simulink model "tyreModelSimu"  (R2020b)
settings: Solver=VariableStepAuto  StartTime=0.0  StopTime=10.0  RelTol=1e-3
values from neighbouring files (symbols this model uses):
  h = 0.3    [Copy_of_model1.m]    (also in model1.m; test.m; tyreModel.m)
  l = lf+lr    (= 2)    [Copy_of_model1.m]    (also in model1.m; test.m = 1.5; tyreModel.m = 1.5)
  lf = 1    [Copy_of_model1.m]    (also in model1.m; test.m; tyreModel.m)
  lr = 1    [Copy_of_model1.m]    (also in model1.m; test.m = 0.5; tyreModel.m = 0.5)
  m = 200    [Copy_of_model1.m]    (also in model1.m; test.m; tyreModel.m)
  rsd = 0.25    [Copy_of_model1.m]    (also in model1.m; test.m; tyreModel.m)
  s1 = 0.5    [Copy_of_model1.m]    (also in model1.m; test.m; tyreModel.m = 1)
  s2 = 0    [Copy_of_model1.m]    (also in model1.m; test.m; tyreModel.m)
undefined symbols (not defined in the file or in its folder): p
libraries: vrlib x3
settings Model: Creator=picku  LastModifiedBy=picku

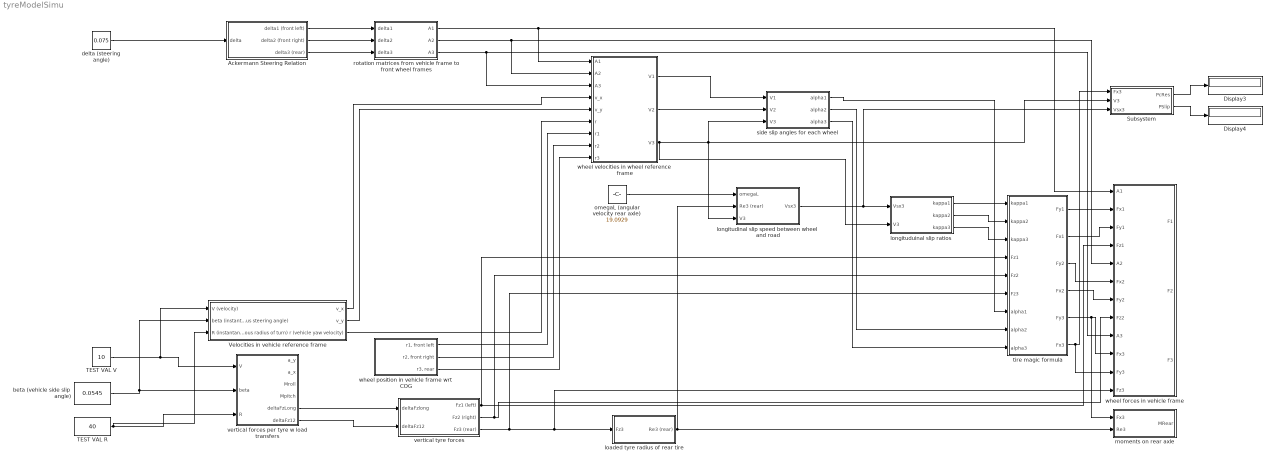
== system tyreModelSimu ==
  Ackermann Steering Relation : Subsystem
  Display3 : Display
  Display4 : Display
  Subsystem : Subsystem
  TEST VAL R : Constant  Value=40
  TEST VAL V : Constant  Value=10
  Velocities in vehicle reference frame : Subsystem
  beta (vehicle side slip angle) : Constant  Value=0.0545
  delta (steering angle) : Constant  Value=0.075
  loaded tyre radius of rear tire : Subsystem
  longitudinal slip speed between wheel and road : Subsystem
  longituduinal slip ratios : Subsystem
  moments on rear axle : Subsystem
  omegaL (angular velocity rear axle) : Constant  Value=19.0929
  rotation matrices from vehicle frame to front wheel frames : Subsystem
  side slip angles for each wheel : Subsystem
  tire magic formula : Subsystem
  vertical forces per tyre w load transfers : Subsystem
  vertical tyre forces : Subsystem
  wheel forces in vehicle frame : Subsystem
  wheel position in vehicle frame wrt COG : Subsystem
  wheel velocities in wheel reference frame : Subsystem
  wires:
  tire magic formula/6("Fx3 ") -> Subsystem/1(Fx3), wheel forces in vehicle frame/11(Fy3)
  longituduinal slip ratios/3(kappa3) -> tire magic formula/3(kappa3)
  tire magic formula/5(Fy3) -> wheel forces in vehicle frame/10(Fx3), moments on rear axle/1(Fx3)
  side slip angles for each wheel/3(alpha3) -> tire magic formula/9(alpha3)
  side slip angles for each wheel/1(alpha1) -> tire magic formula/7(alpha1)
  side slip angles for each wheel/2(alpha2) -> tire magic formula/8(alpha2)
  vertical tyre forces/1(Fz1 (left)) -> tire magic formula/4(Fz1), wheel forces in vehicle frame/4(Fz1)
  tire magic formula/1(Fy1) -> wheel forces in vehicle frame/2(Fx1)
  tire magic formula/2(Fx1) -> wheel forces in vehicle frame/3(Fy1)
  vertical tyre forces/2(Fz2 (right)) -> tire magic formula/5(Fz2), wheel forces in vehicle frame/8(Fz2)
  longituduinal slip ratios/1(kappa1) -> tire magic formula/1(kappa1)
  tire magic formula/4(Fx2) -> wheel forces in vehicle frame/7(Fy2)
  longituduinal slip ratios/2(kappa2) -> tire magic formula/2(kappa2)
  tire magic formula/3(Fy2) -> wheel forces in vehicle frame/6(Fx2)
  vertical tyre forces/3(Fz3 (rear)) -> loaded tyre radius of rear tire/1(Fz3), wheel forces in vehicle frame/12(Fz3), tire magic formula/6(Fz3)
  loaded tyre radius of rear tire/1(Re3 (rear)) -> moments on rear axle/2(Re3), longitudinal slip speed between wheel and road/2(Re3 (rear))
  wheel velocities in wheel reference frame/2(V2) -> side slip angles for each wheel/2(V2)
  longitudinal slip speed between wheel and road/1(Vsx3) -> Subsystem/3(Vsx3), longituduinal slip ratios/1(Vsx3)
  rotation matrices from vehicle frame to front wheel frames/3(A3) -> wheel velocities in wheel reference frame/3(A3), wheel forces in vehicle frame/9(A3)
  wheel position in vehicle frame wrt COG/2("r2, front right") -> wheel velocities in wheel reference frame/8(r2)
  vertical forces per tyre w load transfers/5(deltaFzLong) -> vertical tyre forces/1(deltaFzlong)
  omegaL (angular velocity rear axle)/1 -> longitudinal slip speed between wheel and road/1(omegaL)
  wheel position in vehicle frame wrt COG/3("r3, rear") -> wheel velocities in wheel reference frame/9(r3)
  wheel velocities in wheel reference frame/1(V1) -> side slip angles for each wheel/1(V1)
  vertical forces per tyre w load transfers/6(deltaFz12) -> vertical tyre forces/2(deltaFz12)
  Ackermann Steering Relation/1(delta1 (front left)) -> rotation matrices from vehicle frame to front wheel frames/1(delta1)
  wheel position in vehicle frame wrt COG/1("r1, front left") -> wheel velocities in wheel reference frame/7(r1)
  TEST VAL V/1 -> Velocities in vehicle reference frame/1(V (velocity)), vertical forces per tyre w load transfers/1(V)
  Velocities in vehicle reference frame/3(r (vehicle yaw velocity)) -> wheel velocities in wheel reference frame/6(r)
  rotation matrices from vehicle frame to front wheel frames/2(A2) -> wheel velocities in wheel reference frame/2(A2), wheel forces in vehicle frame/5(A2)
  wheel velocities in wheel reference frame/3(V3) -> side slip angles for each wheel/3(V3), Subsystem/2(V3), longitudinal slip speed between wheel and road/3(V3), longituduinal slip ratios/2(V3)
  Velocities in vehicle reference frame/1(v_x) -> wheel velocities in wheel reference frame/4(v_x)
  Velocities in vehicle reference frame/2(v_y) -> wheel velocities in wheel reference frame/5(v_y)
  rotation matrices from vehicle frame to front wheel frames/1(A1) -> wheel velocities in wheel reference frame/1(A1), wheel forces in vehicle frame/1(A1)
  Ackermann Steering Relation/3(delta3 (rear)) -> rotation matrices from vehicle frame to front wheel frames/3(delta3)
  Ackermann Steering Relation/2(delta2 (front right)) -> rotation matrices from vehicle frame to front wheel frames/2(delta2)
  delta (steering angle)/1 -> Ackermann Steering Relation/1(delta)
  TEST VAL R/1 -> Velocities in vehicle reference frame/3(R (instantaneous radius of turn)), vertical forces per tyre w load transfers/3(R)
  beta (vehicle side slip angle)/1 -> Velocities in vehicle reference frame/2(beta (instantaneous steering angle)), vertical forces per tyre w load transfers/2(beta)
  Subsystem/1(PcRes) -> Display3/1
  Subsystem/2(PSlip) -> Display4/1

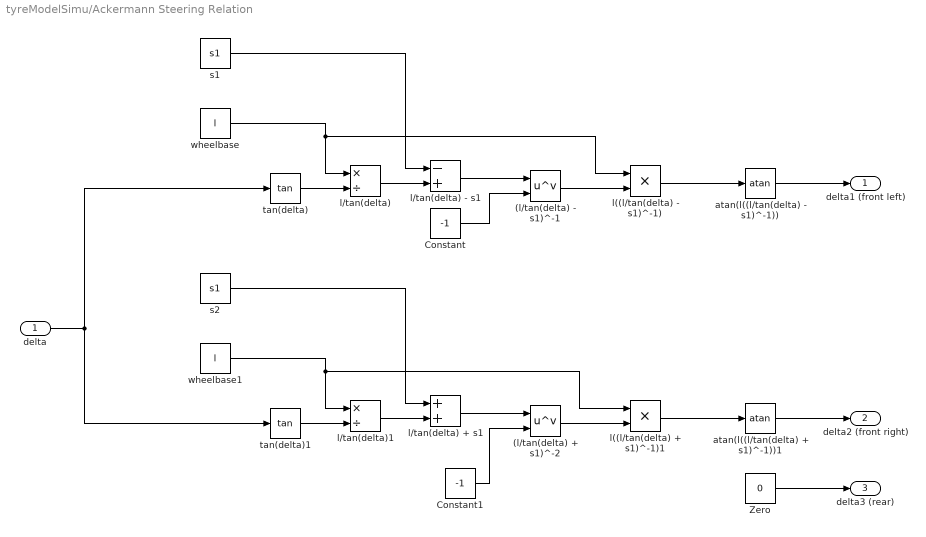
== system tyreModelSimu/Ackermann Steering Relation ==
  delta : Inport
  (l/tan(delta) + s1)^-2 : Math  Operator=pow  SaturateOnIntegerOverflow=on
  (l/tan(delta) - s1)^-1 : Math  Operator=pow  SaturateOnIntegerOverflow=on
  Constant : Constant  Value=-1
  Constant1 : Constant  Value=-1
  Zero : Constant  Value=0  OutDataTypeStr=Inherit: Inherit via back propagation
  atan(l((l/tan(delta) + s1)^-1))1 : Trigonometry  Operator=atan
  atan(l((l/tan(delta) - s1)^-1)) : Trigonometry  Operator=atan
  l((l/tan(delta) + s1)^-1)1 : Product
  l((l/tan(delta) - s1)^-1) : Product
  l/tan(delta) : Product  Inputs=*/
  l/tan(delta) + s1 : Sum
  l/tan(delta) - s1 : Sum  Inputs=-+
  l/tan(delta)1 : Product  Inputs=*/
  s1 : Constant  Value=s1
  s2 : Constant  Value=s1
  tan(delta) : Trigonometry  Operator=tan
  tan(delta)1 : Trigonometry  Operator=tan
  wheelbase : Constant  Value=l
  wheelbase1 : Constant  Value=l
  delta1 (front left) : Outport
  delta2 (front right) : Outport  Port=2
  delta3 (rear) : Outport  Port=3
  wires:
  tan(delta)/1 -> l/tan(delta)/2
  wheelbase/1 -> l((l/tan(delta) - s1)^-1)/1, l/tan(delta)/1
  l/tan(delta)/1 -> l/tan(delta) - s1/2
  s1/1 -> l/tan(delta) - s1/1
  l/tan(delta) - s1/1 -> (l/tan(delta) - s1)^-1/1
  Constant/1 -> (l/tan(delta) - s1)^-1/2
  (l/tan(delta) - s1)^-1/1 -> l((l/tan(delta) - s1)^-1)/2
  l((l/tan(delta) - s1)^-1)/1 -> atan(l((l/tan(delta) - s1)^-1))/1
  atan(l((l/tan(delta) - s1)^-1))/1 -> delta1 (front left)/1
  Constant1/1 -> (l/tan(delta) + s1)^-2/2
  wheelbase1/1 -> l((l/tan(delta) + s1)^-1)1/1, l/tan(delta)1/1
  tan(delta)1/1 -> l/tan(delta)1/2
  (l/tan(delta) + s1)^-2/1 -> l((l/tan(delta) + s1)^-1)1/2
  delta/1 -> tan(delta)1/1, tan(delta)/1
  l/tan(delta) + s1/1 -> (l/tan(delta) + s1)^-2/1
  l/tan(delta)1/1 -> l/tan(delta) + s1/2
  atan(l((l/tan(delta) + s1)^-1))1/1 -> delta2 (front right)/1
  l((l/tan(delta) + s1)^-1)1/1 -> atan(l((l/tan(delta) + s1)^-1))1/1
  s2/1 -> l/tan(delta) + s1/1
  Zero/1 -> delta3 (rear)/1

== system tyreModelSimu/Subsystem ==
  Fx3 : Inport
  V3 : Inport  Port=2
  Vsx3 : Inport  Port=3
  Demux : Demux  Outputs=3
  Product : Product
  Product1 : Product
  PcRes : Outport
  PSlip : Outport  Port=2
  wires:
  V3/1 -> Demux/1
  Demux/1 -> Product/2
  Fx3/1 -> Product1/2, Product/1
  Product/1 -> PcRes/1
  Vsx3/1 -> Product1/1
  Product1/1 -> PSlip/1

== system tyreModelSimu/Velocities in vehicle reference frame ==
  V (velocity) : Inport
  beta (instantaneous steering angle) : Inport  Port=2
  R (instantaneous radius of turn) : Inport  Port=3
  -V*sin(beta) : Product
  -sin(beta) : UnaryMinus
  Divide : Product  Inputs=*/
  V*cos(beta) : Product
  cos(beta) : Trigonometry  Operator=cos
  sin(beta) : Trigonometry
  v_x : Outport
  v_y : Outport  Port=2
  r (vehicle yaw velocity) : Outport  Port=3
  wires:
  beta (instantaneous steering angle)/1 -> sin(beta)/1, cos(beta)/1
  sin(beta)/1 -> -sin(beta)/1
  -sin(beta)/1 -> -V*sin(beta)/2
  V (velocity)/1 -> Divide/1, V*cos(beta)/1, -V*sin(beta)/1
  cos(beta)/1 -> V*cos(beta)/2
  -V*sin(beta)/1 -> v_y/1
  V*cos(beta)/1 -> v_x/1
  R (instantaneous radius of turn)/1 -> Divide/2
  Divide/1 -> r (vehicle yaw velocity)/1

== system tyreModelSimu/loaded tyre radius of rear tire ==
  Fz3 : Inport
  Display : Display
  Divide : Product  Inputs=*/
  Subtract : Sum  Inputs=-+
  free tyre radius : Constant  Value=p.tyre1.R0
  tyre vertical stiffness : Constant  Value=p.tyre1.kz
  Re3 (rear) : Outport
  wires:
  tyre vertical stiffness/1 -> Divide/2
  Fz3/1 -> Display/1, Divide/1
  Divide/1 -> Subtract/1
  free tyre radius/1 -> Subtract/2
  Subtract/1 -> Re3 (rear)/1

== system tyreModelSimu/longitudinal slip speed between wheel and road ==
  omegaL : Inport
  Re3 (rear) : Inport  Port=2
  V3 : Inport  Port=3
  Demux : Demux  Outputs=3
  Display{,1..3} (4 alike) : Display
  Product : Product
  Subtract : Sum  Inputs=-+
  Unary Minus : UnaryMinus
  Vsx3 : Outport
  wires:
  V3/1 -> Display2/1, Demux/1
  omegaL/1 -> Display/1, Product/1
  Re3 (rear)/1 -> Display1/1, Product/2
  Product/1 -> Subtract/1
  Demux/1 -> Subtract/2
  Subtract/1 -> Unary Minus/1
  Unary Minus/1 -> Display3/1, Vsx3/1

== system tyreModelSimu/longituduinal slip ratios ==
  Vsx3 : Inport
  V3 : Inport  Port=2
  Abs : Abs
  Demux : Demux  Outputs=3
  Divide : Product  Inputs=*/
  Zero : Constant  Value=0  OutDataTypeStr=Inherit: Inherit via back propagation
  kappa1 : Outport
  kappa2 : Outport  Port=2
  kappa3 : Outport  Port=3
  wires:
  Zero/1 -> kappa2/1, kappa1/1
  V3/1 -> Demux/1
  Demux/1 -> Abs/1
  Abs/1 -> Divide/2
  Vsx3/1 -> Divide/1
  Divide/1 -> kappa3/1

== system tyreModelSimu/moments on rear axle ==
  Fx3 : Inport
  Re3 : Inport  Port=2
  Product : Product
  MRear : Outport
  wires:
  Re3/1 -> Product/2
  Fx3/1 -> Product/1
  Product/1 -> MRear/1

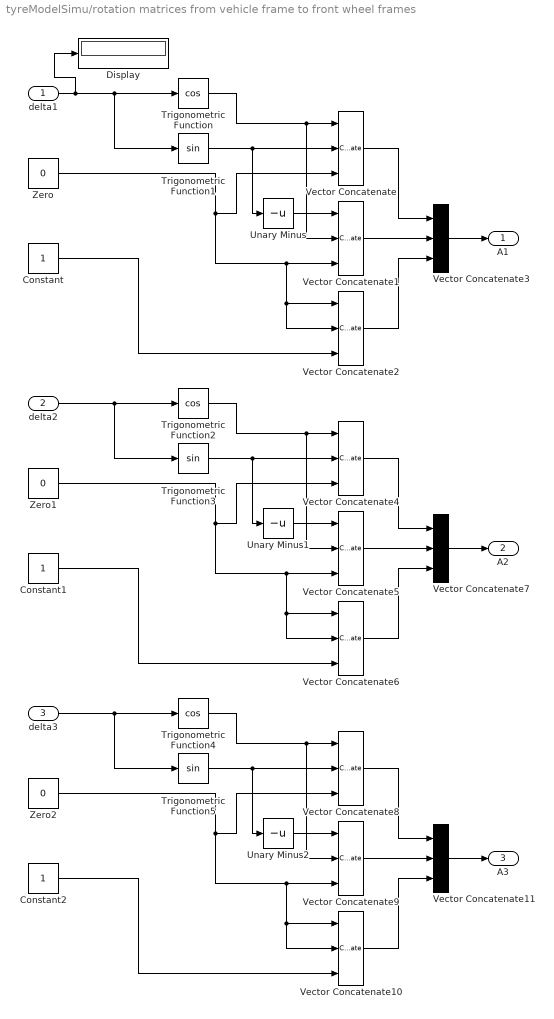
== system tyreModelSimu/rotation matrices from vehicle frame to front wheel frames ==
  delta1 : Inport
  delta2 : Inport  Port=2
  delta3 : Inport  Port=3
  Constant : Constant
  Constant1 : Constant
  Constant2 : Constant
  Display : Display
  Trigonometric Function : Trigonometry  Operator=cos
  Trigonometric Function1 : Trigonometry
  Trigonometric Function2 : Trigonometry  Operator=cos
  Trigonometric Function3 : Trigonometry
  Trigonometric Function4 : Trigonometry  Operator=cos
  Trigonometric Function5 : Trigonometry
  Unary Minus : UnaryMinus
  Unary Minus1 : UnaryMinus
  Unary Minus2 : UnaryMinus
  Vector Concatenate{,1..2,4..6,8..10} (9 alike) : Concatenate  NumInputs=3  Mode=Multidimensional array  ConcatenateDimension=2
  Vector Concatenate11 : Concatenate  NumInputs=3  Mode=Multidimensional array
  Vector Concatenate3 : Concatenate  NumInputs=3  Mode=Multidimensional array
  Vector Concatenate7 : Concatenate  NumInputs=3  Mode=Multidimensional array
  Zero : Constant  Value=0  OutDataTypeStr=Inherit: Inherit via back propagation
  Zero1 : Constant  Value=0  OutDataTypeStr=Inherit: Inherit via back propagation
  Zero2 : Constant  Value=0  OutDataTypeStr=Inherit: Inherit via back propagation
  A1 : Outport
  A2 : Outport  Port=2
  A3 : Outport  Port=3
  wires:
  delta1/1 -> Display/1, Trigonometric Function1/1, Trigonometric Function/1
  Trigonometric Function/1 -> Vector Concatenate1/2, Vector Concatenate/1
  Trigonometric Function1/1 -> Unary Minus/1, Vector Concatenate/2
  Zero/1 -> Vector Concatenate2/2, Vector Concatenate2/1, Vector Concatenate1/3, Vector Concatenate/3
  Unary Minus/1 -> Vector Concatenate1/1
  Constant/1 -> Vector Concatenate2/3
  Vector Concatenate/1 -> Vector Concatenate3/1
  Vector Concatenate1/1 -> Vector Concatenate3/2
  Vector Concatenate2/1 -> Vector Concatenate3/3
  Vector Concatenate3/1 -> A1/1
  Vector Concatenate7/1 -> A2/1
  Constant1/1 -> Vector Concatenate6/3
  Zero1/1 -> Vector Concatenate6/2, Vector Concatenate6/1, Vector Concatenate5/3, Vector Concatenate4/3
  Vector Concatenate5/1 -> Vector Concatenate7/2
  Vector Concatenate4/1 -> Vector Concatenate7/1
  Trigonometric Function2/1 -> Vector Concatenate5/2, Vector Concatenate4/1
  Trigonometric Function3/1 -> Unary Minus1/1, Vector Concatenate4/2
  delta2/1 -> Trigonometric Function3/1, Trigonometric Function2/1
  Vector Concatenate6/1 -> Vector Concatenate7/3
  Unary Minus1/1 -> Vector Concatenate5/1
  Vector Concatenate11/1 -> A3/1
  Constant2/1 -> Vector Concatenate10/3
  Zero2/1 -> Vector Concatenate10/2, Vector Concatenate10/1, Vector Concatenate9/3, Vector Concatenate8/3
  Vector Concatenate9/1 -> Vector Concatenate11/2
  Vector Concatenate8/1 -> Vector Concatenate11/1
  Trigonometric Function4/1 -> Vector Concatenate9/2, Vector Concatenate8/1
  Trigonometric Function5/1 -> Unary Minus2/1, Vector Concatenate8/2
  delta3/1 -> Trigonometric Function5/1, Trigonometric Function4/1
  Vector Concatenate10/1 -> Vector Concatenate11/3
  Unary Minus2/1 -> Vector Concatenate9/1

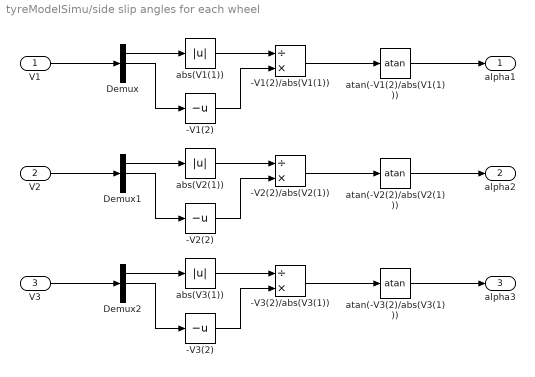
== system tyreModelSimu/side slip angles for each wheel ==
  V1 : Inport
  V2 : Inport  Port=2
  V3 : Inport  Port=3
  -V1(2) : UnaryMinus
  -V1(2)/abs(V1(1)) : Product  Inputs=/*
  -V2(2) : UnaryMinus
  -V2(2)/abs(V2(1)) : Product  Inputs=/*
  -V3(2) : UnaryMinus
  -V3(2)/abs(V3(1)) : Product  Inputs=/*
  Demux : Demux  Outputs=3
  Demux1 : Demux  Outputs=3
  Demux2 : Demux  Outputs=3
  abs(V1(1)) : Abs
  abs(V2(1)) : Abs
  abs(V3(1)) : Abs
  atan(-V1(2)/abs(V1(1))) : Trigonometry  Operator=atan
  atan(-V2(2)/abs(V2(1))) : Trigonometry  Operator=atan
  atan(-V3(2)/abs(V3(1))) : Trigonometry  Operator=atan
  alpha1 : Outport
  alpha2 : Outport  Port=2
  alpha3 : Outport  Port=3
  wires:
  V1/1 -> Demux/1
  Demux/1 -> abs(V1(1))/1
  Demux/2 -> -V1(2)/1
  abs(V1(1))/1 -> -V1(2)/abs(V1(1))/1
  -V1(2)/1 -> -V1(2)/abs(V1(1))/2
  -V1(2)/abs(V1(1))/1 -> atan(-V1(2)/abs(V1(1)))/1
  atan(-V1(2)/abs(V1(1)))/1 -> alpha1/1
  abs(V2(1))/1 -> -V2(2)/abs(V2(1))/1
  -V2(2)/1 -> -V2(2)/abs(V2(1))/2
  Demux1/2 -> -V2(2)/1
  -V2(2)/abs(V2(1))/1 -> atan(-V2(2)/abs(V2(1)))/1
  V2/1 -> Demux1/1
  Demux1/1 -> abs(V2(1))/1
  atan(-V2(2)/abs(V2(1)))/1 -> alpha2/1
  abs(V3(1))/1 -> -V3(2)/abs(V3(1))/1
  -V3(2)/1 -> -V3(2)/abs(V3(1))/2
  Demux2/2 -> -V3(2)/1
  -V3(2)/abs(V3(1))/1 -> atan(-V3(2)/abs(V3(1)))/1
  V3/1 -> Demux2/1
  Demux2/1 -> abs(V3(1))/1
  atan(-V3(2)/abs(V3(1)))/1 -> alpha3/1

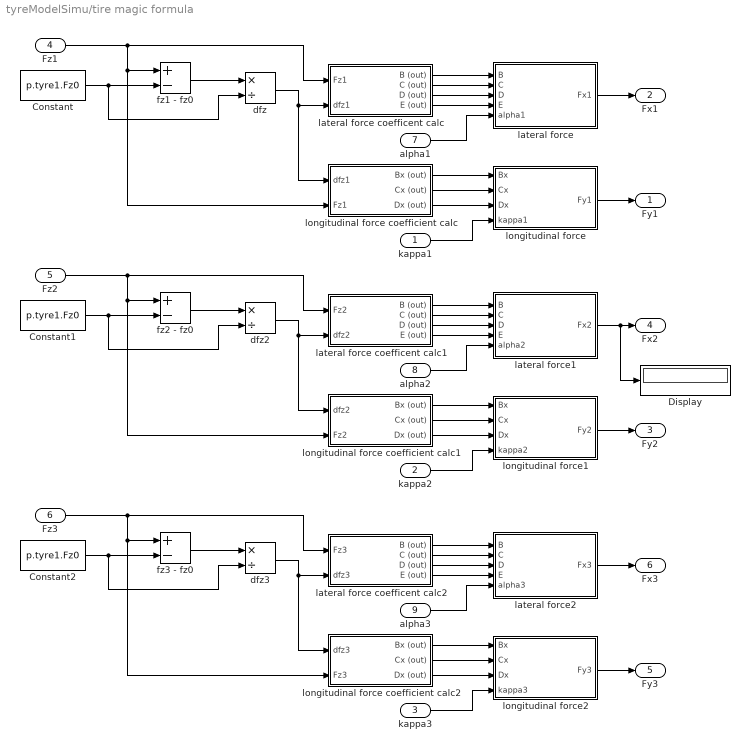
== system tyreModelSimu/tire magic formula ==
  kappa1 : Inport
  kappa2 : Inport  Port=2
  kappa3 : Inport  Port=3
  Fz1 : Inport  Port=4
  Fz2 : Inport  Port=5
  Fz3 : Inport  Port=6
  alpha1 : Inport  Port=7
  alpha2 : Inport  Port=8
  alpha3 : Inport  Port=9
  Constant : Constant  Value=p.tyre1.Fz0
  Constant1 : Constant  Value=p.tyre1.Fz0
  Constant2 : Constant  Value=p.tyre1.Fz0
  Display : Display
  dfz : Product  Inputs=*/
  dfz2 : Product  Inputs=*/
  dfz3 : Product  Inputs=*/
  fz1 - fz0 : Sum  Inputs=+-
  fz2 - fz0 : Sum  Inputs=+-
  fz3 - fz0 : Sum  Inputs=+-
  lateral force : Subsystem
  lateral force coefficent calc : Subsystem
  lateral force coefficent calc1 : Subsystem
  lateral force coefficent calc2 : Subsystem
  lateral force1 : Subsystem
  lateral force2 : Subsystem
  longitudinal force : Subsystem
  longitudinal force coefficient calc : Subsystem
  longitudinal force coefficient calc1 : Subsystem
  longitudinal force coefficient calc2 : Subsystem
  longitudinal force1 : Subsystem
  longitudinal force2 : Subsystem
  Fy1 : Outport
  Fx1 : Outport  Port=2
  Fy2 : Outport  Port=3
  Fx2 : Outport  Port=4
  Fy3 : Outport  Port=5
  "Fx3 " : Outport  Port=6
  wires:
  Fz1/1 -> lateral force coefficent calc/1(Fz1), longitudinal force coefficient calc/2(Fz1), fz1 - fz0/1
  Constant/1 -> fz1 - fz0/2, dfz/2
  fz1 - fz0/1 -> dfz/1
  dfz/1 -> longitudinal force coefficient calc/1(dfz1), lateral force coefficent calc/2(dfz1)
  lateral force coefficent calc/1(B (out)) -> lateral force/1(B)
  lateral force coefficent calc/2(C (out)) -> lateral force/2(C)
  lateral force coefficent calc/3(D (out)) -> lateral force/3(D)
  lateral force coefficent calc/4(E (out)) -> lateral force/4(E)
  alpha1/1 -> lateral force/5(alpha1)
  kappa1/1 -> longitudinal force/4(kappa1)
  longitudinal force coefficient calc/1(Bx (out)) -> longitudinal force/1(Bx)
  longitudinal force coefficient calc/2(Cx (out)) -> longitudinal force/2(Cx)
  longitudinal force coefficient calc/3(Dx (out)) -> longitudinal force/3(Dx)
  lateral force coefficent calc1/3(D (out)) -> lateral force1/3(D)
  lateral force coefficent calc1/4(E (out)) -> lateral force1/4(E)
  lateral force coefficent calc1/2(C (out)) -> lateral force1/2(C)
  longitudinal force coefficient calc1/2(Cx (out)) -> longitudinal force1/2(Cx)
  alpha2/1 -> lateral force1/5(alpha2)
  longitudinal force coefficient calc1/3(Dx (out)) -> longitudinal force1/3(Dx)
  longitudinal force coefficient calc1/1(Bx (out)) -> longitudinal force1/1(Bx)
  Fz2/1 -> lateral force coefficent calc1/1(Fz2), longitudinal force coefficient calc1/2(Fz2), fz2 - fz0/1
  fz2 - fz0/1 -> dfz2/1
  Constant1/1 -> fz2 - fz0/2, dfz2/2
  dfz2/1 -> longitudinal force coefficient calc1/1(dfz2), lateral force coefficent calc1/2(dfz2)
  kappa2/1 -> longitudinal force1/4(kappa2)
  lateral force coefficent calc1/1(B (out)) -> lateral force1/1(B)
  lateral force coefficent calc2/3(D (out)) -> lateral force2/3(D)
  lateral force coefficent calc2/4(E (out)) -> lateral force2/4(E)
  lateral force coefficent calc2/2(C (out)) -> lateral force2/2(C)
  longitudinal force coefficient calc2/2(Cx (out)) -> longitudinal force2/2(Cx)
  alpha3/1 -> lateral force2/5(alpha3)
  longitudinal force coefficient calc2/3(Dx (out)) -> longitudinal force2/3(Dx)
  longitudinal force coefficient calc2/1(Bx (out)) -> longitudinal force2/1(Bx)
  Fz3/1 -> lateral force coefficent calc2/1(Fz3), longitudinal force coefficient calc2/2(Fz3), fz3 - fz0/1
  fz3 - fz0/1 -> dfz3/1
  Constant2/1 -> fz3 - fz0/2, dfz3/2
  dfz3/1 -> longitudinal force coefficient calc2/1(dfz3), lateral force coefficent calc2/2(dfz3)
  kappa3/1 -> longitudinal force2/4(kappa3)
  lateral force coefficent calc2/1(B (out)) -> lateral force2/1(B)
  longitudinal force/1(Fy1) -> Fy1/1
  lateral force/1(Fx1) -> Fx1/1
  longitudinal force1/1(Fy2) -> Fy2/1
  lateral force1/1(Fx2) -> Display/1, Fx2/1
  longitudinal force2/1(Fy3) -> Fy3/1
  lateral force2/1(Fx3) -> "Fx3 "/1

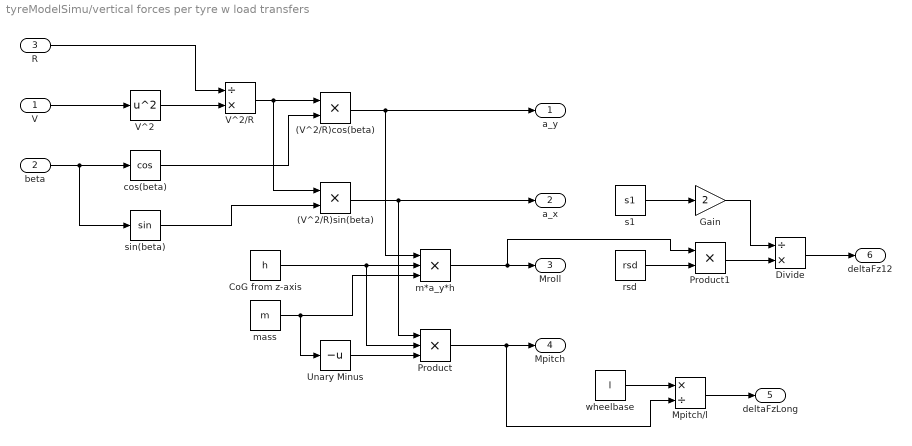
== system tyreModelSimu/vertical forces per tyre w load transfers ==
  V : Inport
  beta : Inport  Port=2
  R : Inport  Port=3
  (V^2/R)cos(beta) : Product
  (V^2/R)sin(beta) : Product
  CoG from z-axis : Constant  Value=h
  Divide : Product  Inputs=/*
  Gain : Gain  Gain=2
  Mpitch/l : Product  Inputs=*/
  Product : Product  Inputs=3
  Product1 : Product
  Unary Minus : UnaryMinus
  V^2 : Math  Operator=square  SaturateOnIntegerOverflow=on
  V^2/R : Product  Inputs=/*
  cos(beta) : Trigonometry  Operator=cos
  m*a_y*h : Product  Inputs=3
  mass : Constant  Value=m
  rsd : Constant  Value=rsd
  s1 : Constant  Value=s1
  sin(beta) : Trigonometry
  wheelbase : Constant  Value=l
  a_y : Outport
  a_x : Outport  Port=2
  Mroll : Outport  Port=3
  Mpitch : Outport  Port=4
  deltaFzLong : Outport  Port=5
  deltaFz12 : Outport  Port=6
  wires:
  V/1 -> V^2/1
  R/1 -> V^2/R/1
  V^2/1 -> V^2/R/2
  beta/1 -> sin(beta)/1, cos(beta)/1
  V^2/R/1 -> (V^2/R)sin(beta)/1, (V^2/R)cos(beta)/1
  cos(beta)/1 -> (V^2/R)cos(beta)/2
  (V^2/R)cos(beta)/1 -> m*a_y*h/1, a_y/1
  sin(beta)/1 -> (V^2/R)sin(beta)/2
  (V^2/R)sin(beta)/1 -> Product/1, a_x/1
  CoG from z-axis/1 -> Product/2, m*a_y*h/2
  mass/1 -> Unary Minus/1, m*a_y*h/3
  m*a_y*h/1 -> Product1/1, Mroll/1
  Product/1 -> Mpitch/l/2, Mpitch/1
  Unary Minus/1 -> Product/3
  wheelbase/1 -> Mpitch/l/1
  Mpitch/l/1 -> deltaFzLong/1
  rsd/1 -> Product1/2
  s1/1 -> Gain/1
  Product1/1 -> Divide/2
  Gain/1 -> Divide/1
  Divide/1 -> deltaFz12/1

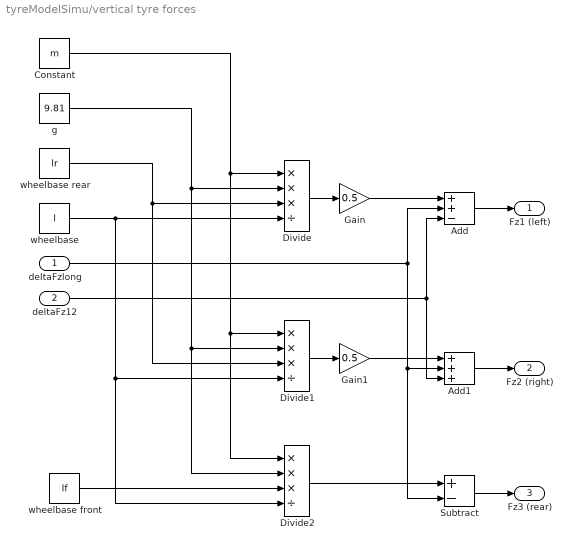
== system tyreModelSimu/vertical tyre forces ==
  deltaFzlong : Inport
  deltaFz12 : Inport  Port=2
  Add : Sum  Inputs=++-
  Add1 : Sum  Inputs=+++
  Constant : Constant  Value=m
  Divide : Product  Inputs=***/
  Divide1 : Product  Inputs=***/
  Divide2 : Product  Inputs=***/
  Gain : Gain  Gain=0.5
  Gain1 : Gain  Gain=0.5
  Subtract : Sum  Inputs=+-
  g : Constant  Value=9.81
  wheelbase : Constant  Value=l
  wheelbase front : Constant  Value=lf
  wheelbase rear : Constant  Value=lr
  Fz1 (left) : Outport
  Fz2 (right) : Outport  Port=2
  Fz3 (rear) : Outport  Port=3
  wires:
  Constant/1 -> Divide2/1, Divide1/1, Divide/1
  g/1 -> Divide2/2, Divide1/2, Divide/2
  wheelbase rear/1 -> Divide1/3, Divide/3
  wheelbase/1 -> Divide2/4, Divide1/4, Divide/4
  Divide/1 -> Gain/1
  Gain/1 -> Add/1
  deltaFzlong/1 -> Subtract/2, Add1/2, Add/2
  deltaFz12/1 -> Add1/3, Add/3
  Add/1 -> Fz1 (left)/1
  Gain1/1 -> Add1/1
  Add1/1 -> Fz2 (right)/1
  Divide1/1 -> Gain1/1
  wheelbase front/1 -> Divide2/3
  Divide2/1 -> Subtract/1
  Subtract/1 -> Fz3 (rear)/1

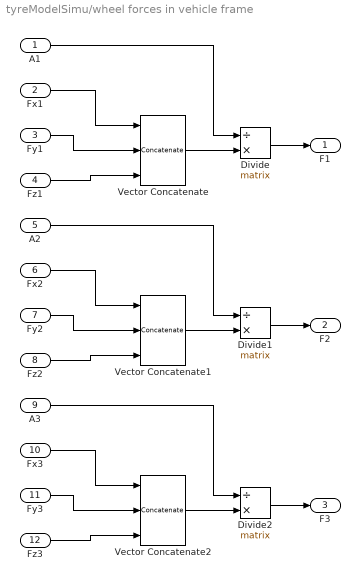
== system tyreModelSimu/wheel forces in vehicle frame ==
  A1 : Inport
  Fx1 : Inport  Port=2
  Fy1 : Inport  Port=3
  Fz1 : Inport  Port=4
  A2 : Inport  Port=5
  Fx2 : Inport  Port=6
  Fy2 : Inport  Port=7
  Fz2 : Inport  Port=8
  A3 : Inport  Port=9
  Fx3 : Inport  Port=10
  Fy3 : Inport  Port=11
  Fz3 : Inport  Port=12
  Divide : Product  Inputs=/*  Multiplication=Matrix(*)
  Divide1 : Product  Inputs=/*  Multiplication=Matrix(*)
  Divide2 : Product  Inputs=/*  Multiplication=Matrix(*)
  Vector Concatenate : Concatenate  NumInputs=3  Mode=Multidimensional array
  Vector Concatenate1 : Concatenate  NumInputs=3  Mode=Multidimensional array
  Vector Concatenate2 : Concatenate  NumInputs=3  Mode=Multidimensional array
  F1 : Outport
  F2 : Outport  Port=2
  F3 : Outport  Port=3
  wires:
  Fx1/1 -> Vector Concatenate/1
  Fy1/1 -> Vector Concatenate/2
  Fz1/1 -> Vector Concatenate/3
  Vector Concatenate/1 -> Divide/2
  A1/1 -> Divide/1
  Divide/1 -> F1/1
  Fz2/1 -> Vector Concatenate1/3
  Divide1/1 -> F2/1
  A2/1 -> Divide1/1
  Fy2/1 -> Vector Concatenate1/2
  Vector Concatenate1/1 -> Divide1/2
  Fx2/1 -> Vector Concatenate1/1
  Fz3/1 -> Vector Concatenate2/3
  Divide2/1 -> F3/1
  A3/1 -> Divide2/1
  Fy3/1 -> Vector Concatenate2/2
  Vector Concatenate2/1 -> Divide2/2
  Fx3/1 -> Vector Concatenate2/1

== system tyreModelSimu/wheel position in vehicle frame wrt COG ==
  Unary Minus : UnaryMinus
  Unary Minus1 : UnaryMinus
  Zero : Constant  Value=0  OutDataTypeStr=Inherit: Inherit via back propagation
  front lateral axle length / 2 : Constant  Value=s1
  r1 front left : Concatenate  NumInputs=3  Mode=Multidimensional array
  r2 front right : Concatenate  NumInputs=3  Mode=Multidimensional array
  r3 rear : Concatenate  NumInputs=3  Mode=Multidimensional array
  rear lateral axle length : Constant  Value=s2
  wheelbase front : Constant  Value=lf
  wheelbase rear : Constant  Value=lr
  "r1, front left" : Outport
  "r2, front right" : Outport  Port=2
  "r3, rear" : Outport  Port=3
  wires:
  wheelbase front/1 -> r2 front right/1, r1 front left/1
  r1 front left/1 -> "r1, front left"/1
  front lateral axle length / 2/1 -> r1 front left/2, Unary Minus/1
  Zero/1 -> r2 front right/3, r3 rear/3, r1 front left/3
  Unary Minus/1 -> r2 front right/2
  r2 front right/1 -> "r2, front right"/1
  Unary Minus1/1 -> r3 rear/1
  wheelbase rear/1 -> Unary Minus1/1
  rear lateral axle length/1 -> r3 rear/2
  r3 rear/1 -> "r3, rear"/1

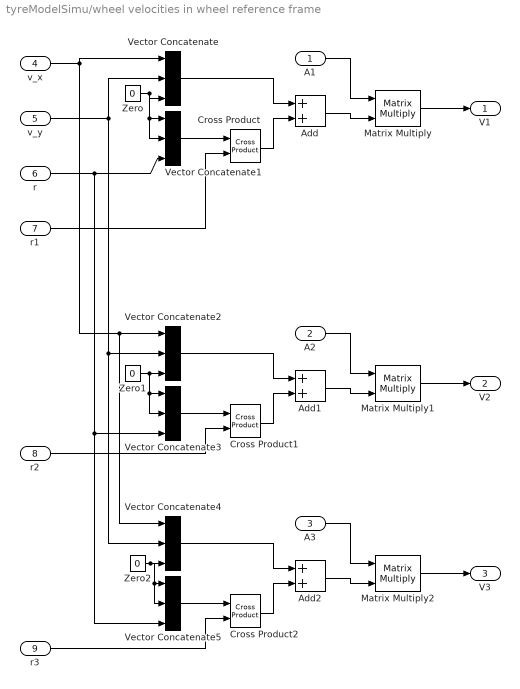
== system tyreModelSimu/wheel velocities in wheel reference frame ==
  A1 : Inport
  A2 : Inport  Port=2
  A3 : Inport  Port=3
  v_x : Inport  Port=4
  v_y : Inport  Port=5
  r : Inport  Port=6
  r1 : Inport  Port=7
  r2 : Inport  Port=8
  r3 : Inport  Port=9
  Add : Sum
  Add1 : Sum
  Add2 : Sum
  Cross Product : vrlib/Utilities/Cross Product
  Cross Product1 : vrlib/Utilities/Cross Product
  Cross Product2 : vrlib/Utilities/Cross Product
  Matrix Multiply : Product  Multiplication=Matrix(*)
  Matrix Multiply1 : Product  Multiplication=Matrix(*)
  Matrix Multiply2 : Product  Multiplication=Matrix(*)
  Vector Concatenate{,1..5} (6 alike) : Concatenate  NumInputs=3  Mode=Multidimensional array
  Zero : Constant  Value=0  OutDataTypeStr=Inherit: Inherit via back propagation
  Zero1 : Constant  Value=0  OutDataTypeStr=Inherit: Inherit via back propagation
  Zero2 : Constant  Value=0  OutDataTypeStr=Inherit: Inherit via back propagation
  V1 : Outport
  V2 : Outport  Port=2
  V3 : Outport  Port=3
  wires:
  Zero/1 -> Vector Concatenate1/2, Vector Concatenate1/1, Vector Concatenate/3
  Vector Concatenate1/1 -> Cross Product/1
  r1/1 -> Cross Product/2
  Cross Product/1 -> Add/2
  Vector Concatenate/1 -> Add/1
  Add/1 -> Matrix Multiply/2
  A1/1 -> Matrix Multiply/1
  Matrix Multiply/1 -> V1/1
  A2/1 -> Matrix Multiply1/1
  Matrix Multiply1/1 -> V2/1
  r2/1 -> Cross Product1/2
  Cross Product1/1 -> Add1/2
  r/1 -> Vector Concatenate1/3, Vector Concatenate5/3, Vector Concatenate3/3
  Vector Concatenate3/1 -> Cross Product1/1
  v_y/1 -> Vector Concatenate4/2, Vector Concatenate2/2, Vector Concatenate/2
  Zero1/1 -> Vector Concatenate2/3, Vector Concatenate3/2, Vector Concatenate3/1
  Add1/1 -> Matrix Multiply1/2
  Vector Concatenate2/1 -> Add1/1
  v_x/1 -> Vector Concatenate4/1, Vector Concatenate2/1, Vector Concatenate/1
  Vector Concatenate4/1 -> Add2/1
  Cross Product2/1 -> Add2/2
  Matrix Multiply2/1 -> V3/1
  Vector Concatenate5/1 -> Cross Product2/1
  Add2/1 -> Matrix Multiply2/2
  Zero2/1 -> Vector Concatenate5/1, Vector Concatenate5/2, Vector Concatenate4/3
  r3/1 -> Cross Product2/2
  A3/1 -> Matrix Multiply2/1

== system tyreModelSimu/tire magic formula/lateral force ==
  B : Inport
  C : Inport  Port=2
  D : Inport  Port=3
  E : Inport  Port=4
  alpha1 : Inport  Port=5
  " " : Product
  Add : Sum
  Constant : Constant
  Product : Product
  Product1 : Product
  Product2 : Product  Inputs=3
  Product3 : Product
  Subtract : Sum  Inputs=+-
  Trigonometric Function : Trigonometry  Operator=atan
  Trigonometric Function1 : Trigonometry  Operator=atan
  Trigonometric Function2 : Trigonometry
  Fx1 : Outport
  wires:
  alpha1/1 -> Subtract/2, Product2/2, Product/2
  B/1 -> Product/1, Product2/3
  Product/1 -> Trigonometric Function/1
  Trigonometric Function/1 -> Product1/2
  E/1 -> Product1/1
  Product1/1 -> Add/2
  Constant/1 -> Subtract/1
  Subtract/1 -> Product2/1
  Product2/1 -> Add/1
  Add/1 -> Trigonometric Function1/1
  Trigonometric Function1/1 -> Product3/2
  C/1 -> Product3/1
  Product3/1 -> Trigonometric Function2/1
  Trigonometric Function2/1 -> " "/2
  D/1 -> " "/1
  " "/1 -> Fx1/1

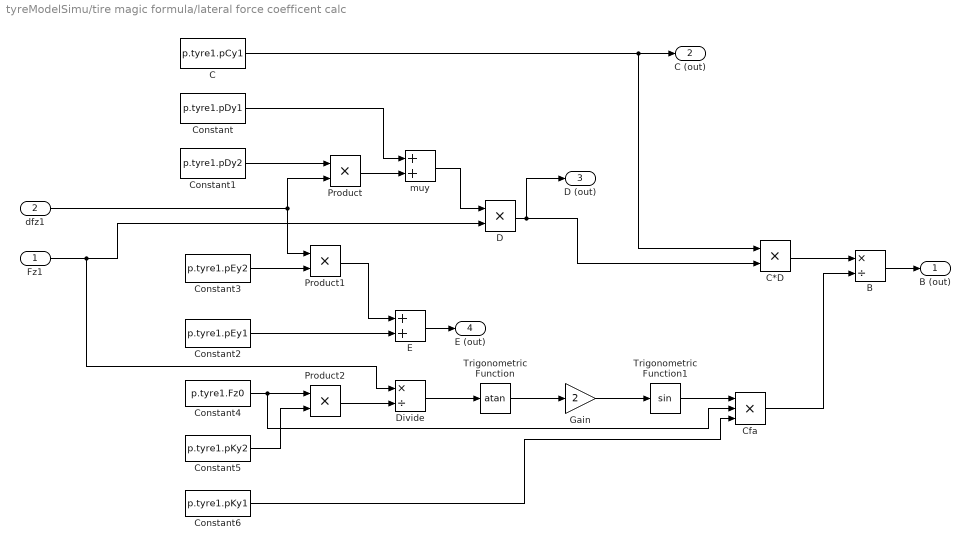
== system tyreModelSimu/tire magic formula/lateral force coefficent calc ==
  Fz1 : Inport
  dfz1 : Inport  Port=2
  B : Product  Inputs=*/
  C : Constant  Value=p.tyre1.pCy1
  C*D : Product
  Cfa : Product  Inputs=3
  Constant : Constant  Value=p.tyre1.pDy1
  Constant1 : Constant  Value=p.tyre1.pDy2
  Constant2 : Constant  Value=p.tyre1.pEy1
  Constant3 : Constant  Value=p.tyre1.pEy2
  Constant4 : Constant  Value=p.tyre1.Fz0
  Constant5 : Constant  Value=p.tyre1.pKy2
  Constant6 : Constant  Value=p.tyre1.pKy1
  D : Product
  Divide : Product  Inputs=*/
  E : Sum
  Gain : Gain  Gain=2
  Product : Product
  Product1 : Product
  Product2 : Product
  Trigonometric Function : Trigonometry  Operator=atan
  Trigonometric Function1 : Trigonometry
  muy : Sum
  B (out) : Outport
  C (out) : Outport  Port=2
  D (out) : Outport  Port=3
  E (out) : Outport  Port=4
  wires:
  dfz1/1 -> Product1/1, Product/2
  Constant1/1 -> Product/1
  Product/1 -> muy/2
  Constant/1 -> muy/1
  Fz1/1 -> Divide/1, D/2
  muy/1 -> D/1
  Constant3/1 -> Product1/2
  Product1/1 -> E/1
  Constant2/1 -> E/2
  Constant4/1 -> Product2/1, Cfa/2
  Constant5/1 -> Product2/2
  Product2/1 -> Divide/2
  Divide/1 -> Trigonometric Function/1
  Trigonometric Function/1 -> Gain/1
  Gain/1 -> Trigonometric Function1/1
  Trigonometric Function1/1 -> Cfa/1
  Constant6/1 -> Cfa/3
  C/1 -> C (out)/1, C*D/1
  D/1 -> D (out)/1, C*D/2
  C*D/1 -> B/1
  Cfa/1 -> B/2
  B/1 -> B (out)/1
  E/1 -> E (out)/1

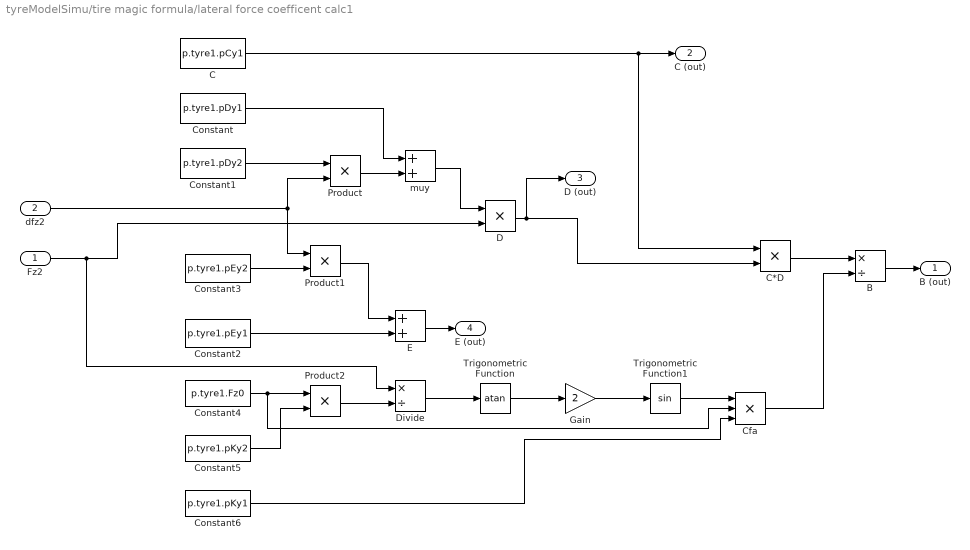
== system tyreModelSimu/tire magic formula/lateral force coefficent calc1 ==
  Fz2 : Inport
  dfz2 : Inport  Port=2
  B : Product  Inputs=*/
  C : Constant  Value=p.tyre1.pCy1
  C*D : Product
  Cfa : Product  Inputs=3
  Constant : Constant  Value=p.tyre1.pDy1
  Constant1 : Constant  Value=p.tyre1.pDy2
  Constant2 : Constant  Value=p.tyre1.pEy1
  Constant3 : Constant  Value=p.tyre1.pEy2
  Constant4 : Constant  Value=p.tyre1.Fz0
  Constant5 : Constant  Value=p.tyre1.pKy2
  Constant6 : Constant  Value=p.tyre1.pKy1
  D : Product
  Divide : Product  Inputs=*/
  E : Sum
  Gain : Gain  Gain=2
  Product : Product
  Product1 : Product
  Product2 : Product
  Trigonometric Function : Trigonometry  Operator=atan
  Trigonometric Function1 : Trigonometry
  muy : Sum
  B (out) : Outport
  C (out) : Outport  Port=2
  D (out) : Outport  Port=3
  E (out) : Outport  Port=4
  wires:
  dfz2/1 -> Product1/1, Product/2
  Constant1/1 -> Product/1
  Product/1 -> muy/2
  Constant/1 -> muy/1
  Fz2/1 -> Divide/1, D/2
  muy/1 -> D/1
  Constant3/1 -> Product1/2
  Product1/1 -> E/1
  Constant2/1 -> E/2
  Constant4/1 -> Product2/1, Cfa/2
  Constant5/1 -> Product2/2
  Product2/1 -> Divide/2
  Divide/1 -> Trigonometric Function/1
  Trigonometric Function/1 -> Gain/1
  Gain/1 -> Trigonometric Function1/1
  Trigonometric Function1/1 -> Cfa/1
  Constant6/1 -> Cfa/3
  C/1 -> C (out)/1, C*D/1
  D/1 -> D (out)/1, C*D/2
  C*D/1 -> B/1
  Cfa/1 -> B/2
  B/1 -> B (out)/1
  E/1 -> E (out)/1

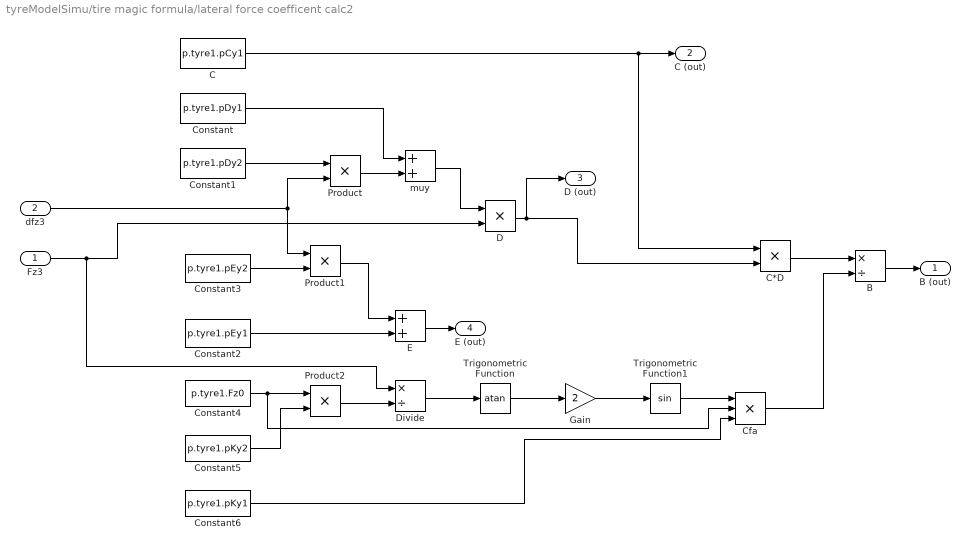
== system tyreModelSimu/tire magic formula/lateral force coefficent calc2 ==
  Fz3 : Inport
  dfz3 : Inport  Port=2
  B : Product  Inputs=*/
  C : Constant  Value=p.tyre1.pCy1
  C*D : Product
  Cfa : Product  Inputs=3
  Constant : Constant  Value=p.tyre1.pDy1
  Constant1 : Constant  Value=p.tyre1.pDy2
  Constant2 : Constant  Value=p.tyre1.pEy1
  Constant3 : Constant  Value=p.tyre1.pEy2
  Constant4 : Constant  Value=p.tyre1.Fz0
  Constant5 : Constant  Value=p.tyre1.pKy2
  Constant6 : Constant  Value=p.tyre1.pKy1
  D : Product
  Divide : Product  Inputs=*/
  E : Sum
  Gain : Gain  Gain=2
  Product : Product
  Product1 : Product
  Product2 : Product
  Trigonometric Function : Trigonometry  Operator=atan
  Trigonometric Function1 : Trigonometry
  muy : Sum
  B (out) : Outport
  C (out) : Outport  Port=2
  D (out) : Outport  Port=3
  E (out) : Outport  Port=4
  wires:
  dfz3/1 -> Product1/1, Product/2
  Constant1/1 -> Product/1
  Product/1 -> muy/2
  Constant/1 -> muy/1
  Fz3/1 -> Divide/1, D/2
  muy/1 -> D/1
  Constant3/1 -> Product1/2
  Product1/1 -> E/1
  Constant2/1 -> E/2
  Constant4/1 -> Product2/1, Cfa/2
  Constant5/1 -> Product2/2
  Product2/1 -> Divide/2
  Divide/1 -> Trigonometric Function/1
  Trigonometric Function/1 -> Gain/1
  Gain/1 -> Trigonometric Function1/1
  Trigonometric Function1/1 -> Cfa/1
  Constant6/1 -> Cfa/3
  C/1 -> C (out)/1, C*D/1
  D/1 -> D (out)/1, C*D/2
  C*D/1 -> B/1
  Cfa/1 -> B/2
  B/1 -> B (out)/1
  E/1 -> E (out)/1

== system tyreModelSimu/tire magic formula/lateral force1 ==
  B : Inport
  C : Inport  Port=2
  D : Inport  Port=3
  E : Inport  Port=4
  alpha2 : Inport  Port=5
  " " : Product
  Add : Sum
  Constant : Constant
  Product : Product
  Product1 : Product
  Product2 : Product  Inputs=3
  Product3 : Product
  Subtract : Sum  Inputs=+-
  Trigonometric Function : Trigonometry  Operator=atan
  Trigonometric Function1 : Trigonometry  Operator=atan
  Trigonometric Function2 : Trigonometry
  Fx2 : Outport
  wires:
  alpha2/1 -> Subtract/2, Product2/2, Product/2
  B/1 -> Product/1, Product2/3
  Product/1 -> Trigonometric Function/1
  Trigonometric Function/1 -> Product1/2
  E/1 -> Product1/1
  Product1/1 -> Add/2
  Constant/1 -> Subtract/1
  Subtract/1 -> Product2/1
  Product2/1 -> Add/1
  Add/1 -> Trigonometric Function1/1
  Trigonometric Function1/1 -> Product3/2
  C/1 -> Product3/1
  Product3/1 -> Trigonometric Function2/1
  Trigonometric Function2/1 -> " "/2
  D/1 -> " "/1
  " "/1 -> Fx2/1

== system tyreModelSimu/tire magic formula/lateral force2 ==
  B : Inport
  C : Inport  Port=2
  D : Inport  Port=3
  E : Inport  Port=4
  alpha3 : Inport  Port=5
  " " : Product
  Add : Sum
  Constant : Constant
  Product : Product
  Product1 : Product
  Product2 : Product  Inputs=3
  Product3 : Product
  Subtract : Sum  Inputs=+-
  Trigonometric Function : Trigonometry  Operator=atan
  Trigonometric Function1 : Trigonometry  Operator=atan
  Trigonometric Function2 : Trigonometry
  Fx3 : Outport
  wires:
  alpha3/1 -> Subtract/2, Product2/2, Product/2
  B/1 -> Product/1, Product2/3
  Product/1 -> Trigonometric Function/1
  Trigonometric Function/1 -> Product1/2
  E/1 -> Product1/1
  Product1/1 -> Add/2
  Constant/1 -> Subtract/1
  Subtract/1 -> Product2/1
  Product2/1 -> Add/1
  Add/1 -> Trigonometric Function1/1
  Trigonometric Function1/1 -> Product3/2
  C/1 -> Product3/1
  Product3/1 -> Trigonometric Function2/1
  Trigonometric Function2/1 -> " "/2
  D/1 -> " "/1
  " "/1 -> Fx3/1

== system tyreModelSimu/tire magic formula/longitudinal force ==
  Bx : Inport
  Cx : Inport  Port=2
  Dx : Inport  Port=3
  kappa1 : Inport  Port=4
  Product : Product
  Product1 : Product
  Product2 : Product
  Subtract : Sum  Inputs=+-
  Subtract1 : Sum  Inputs=+-
  Trigonometric Function : Trigonometry  Operator=atan
  Trigonometric Function1 : Trigonometry  Operator=atan
  Trigonometric Function2 : Trigonometry
  Fy1 : Outport
  wires:
  kappa1/1 -> Product/2
  Bx/1 -> Product/1
  Product/1 -> Subtract1/1, Subtract/1, Trigonometric Function/1
  Trigonometric Function/1 -> Subtract/2
  Subtract/1 -> Subtract1/2
  Subtract1/1 -> Trigonometric Function1/1
  Trigonometric Function1/1 -> Product1/2
  Cx/1 -> Product1/1
  Product1/1 -> Trigonometric Function2/1
  Trigonometric Function2/1 -> Product2/2
  Dx/1 -> Product2/1
  Product2/1 -> Fy1/1

== system tyreModelSimu/tire magic formula/longitudinal force coefficient calc ==
  dfz1 : Inport
  Fz1 : Inport  Port=2
  " " : Constant  Value=p.tyre1.pDx1
  " 1" : Constant  Value=p.tyre1.pDx2
  " 2" : Constant  Value=p.tyre1.pKx1
  Bx : Product  Inputs=/*
  Cx : Constant  Value=p.tyre1.pCx1
  Dx : Product
  Kx : Product
  Product : Product
  Product1 : Product
  mux : Sum
  Bx (out) : Outport
  Cx (out) : Outport  Port=2
  Dx (out) : Outport  Port=3
  wires:
  " 1"/1 -> Product/1
  dfz1/1 -> Product/2
  Product/1 -> mux/2
  " "/1 -> mux/1
  Fz1/1 -> Kx/1, Dx/2
  mux/1 -> Dx/1
  Cx/1 -> Product1/1, Cx (out)/1
  Dx/1 -> Product1/2, Dx (out)/1
  " 2"/1 -> Kx/2
  Kx/1 -> Bx/2
  Product1/1 -> Bx/1
  Bx/1 -> Bx (out)/1

== system tyreModelSimu/tire magic formula/longitudinal force coefficient calc1 ==
  dfz2 : Inport
  Fz2 : Inport  Port=2
  " " : Constant  Value=p.tyre1.pDx1
  " 1" : Constant  Value=p.tyre1.pDx2
  " 2" : Constant  Value=p.tyre1.pKx1
  Bx : Product  Inputs=/*
  Cx : Constant  Value=p.tyre1.pCx1
  Dx : Product
  Kx : Product
  Product : Product
  Product1 : Product
  mux : Sum
  Bx (out) : Outport
  Cx (out) : Outport  Port=2
  Dx (out) : Outport  Port=3
  wires:
  " 1"/1 -> Product/1
  dfz2/1 -> Product/2
  Product/1 -> mux/2
  " "/1 -> mux/1
  Fz2/1 -> Kx/1, Dx/2
  mux/1 -> Dx/1
  Cx/1 -> Product1/1, Cx (out)/1
  Dx/1 -> Product1/2, Dx (out)/1
  " 2"/1 -> Kx/2
  Kx/1 -> Bx/2
  Product1/1 -> Bx/1
  Bx/1 -> Bx (out)/1

== system tyreModelSimu/tire magic formula/longitudinal force coefficient calc2 ==
  dfz3 : Inport
  Fz3 : Inport  Port=2
  " " : Constant  Value=p.tyre1.pDx1
  " 1" : Constant  Value=p.tyre1.pDx2
  " 2" : Constant  Value=p.tyre1.pKx1
  Bx : Product  Inputs=/*
  Cx : Constant  Value=p.tyre1.pCx1
  Dx : Product
  Kx : Product
  Product : Product
  Product1 : Product
  mux : Sum
  Bx (out) : Outport
  Cx (out) : Outport  Port=2
  Dx (out) : Outport  Port=3
  wires:
  " 1"/1 -> Product/1
  dfz3/1 -> Product/2
  Product/1 -> mux/2
  " "/1 -> mux/1
  Fz3/1 -> Kx/1, Dx/2
  mux/1 -> Dx/1
  Cx/1 -> Product1/1, Cx (out)/1
  Dx/1 -> Product1/2, Dx (out)/1
  " 2"/1 -> Kx/2
  Kx/1 -> Bx/2
  Product1/1 -> Bx/1
  Bx/1 -> Bx (out)/1

== system tyreModelSimu/tire magic formula/longitudinal force1 ==
  Bx : Inport
  Cx : Inport  Port=2
  Dx : Inport  Port=3
  kappa2 : Inport  Port=4
  Product : Product
  Product1 : Product
  Product2 : Product
  Subtract : Sum  Inputs=+-
  Subtract1 : Sum  Inputs=+-
  Trigonometric Function : Trigonometry  Operator=atan
  Trigonometric Function1 : Trigonometry  Operator=atan
  Trigonometric Function2 : Trigonometry
  Fy2 : Outport
  wires:
  kappa2/1 -> Product/2
  Bx/1 -> Product/1
  Product/1 -> Subtract1/1, Subtract/1, Trigonometric Function/1
  Trigonometric Function/1 -> Subtract/2
  Subtract/1 -> Subtract1/2
  Subtract1/1 -> Trigonometric Function1/1
  Trigonometric Function1/1 -> Product1/2
  Cx/1 -> Product1/1
  Product1/1 -> Trigonometric Function2/1
  Trigonometric Function2/1 -> Product2/2
  Dx/1 -> Product2/1
  Product2/1 -> Fy2/1

== system tyreModelSimu/tire magic formula/longitudinal force2 ==
  Bx : Inport
  Cx : Inport  Port=2
  Dx : Inport  Port=3
  kappa3 : Inport  Port=4
  Product : Product
  Product1 : Product
  Product2 : Product
  Subtract : Sum  Inputs=+-
  Subtract1 : Sum  Inputs=+-
  Trigonometric Function : Trigonometry  Operator=atan
  Trigonometric Function1 : Trigonometry  Operator=atan
  Trigonometric Function2 : Trigonometry
  Fy3 : Outport
  wires:
  kappa3/1 -> Product/2
  Bx/1 -> Product/1
  Product/1 -> Subtract1/1, Subtract/1, Trigonometric Function/1
  Trigonometric Function/1 -> Subtract/2
  Subtract/1 -> Subtract1/2
  Subtract1/1 -> Trigonometric Function1/1
  Trigonometric Function1/1 -> Product1/2
  Cx/1 -> Product1/1
  Product1/1 -> Trigonometric Function2/1
  Trigonometric Function2/1 -> Product2/2
  Dx/1 -> Product2/1
  Product2/1 -> Fy3/1
